simulink model "model2"  (R2016a)
settings: Solver=VariableStepAuto  StartTime=0.0  StopTime=10.0  RelTol=1e-3
settings Model: Creator=STEM Student  LastModifiedBy=STEM Student

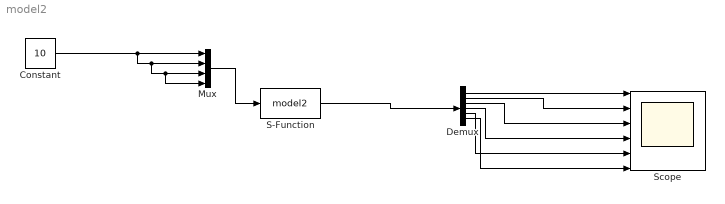
== system model2 ==
  Constant : Constant  Value=10
  Demux : Demux  Outputs=6
  Mux : Mux
  S-Function : S-Function  FunctionName=model2  SFunctionDeploymentMode=off  EnableBusSupport=off
  Scope : Scope  NumInputPorts=6
  wires:
  Constant/1 -> Mux/4, Mux/3, Mux/2, Mux/1
  Mux/1 -> S-Function/1
  S-Function/1 -> Demux/1
  Demux/1 -> Scope/1
  Demux/3 -> Scope/3
  Demux/2 -> Scope/2
  Demux/4 -> Scope/4
  Demux/5 -> Scope/5
  Demux/6 -> Scope/6
